simulink model "MyBattery_RTW"  (Simulink 10.1)
settings: Solver=ode1  StartTime=0.0  StopTime=inf  FixedStep=0.0002  RelTol=1e-3
PreLoadFcn:
  | vehicle = 'Car'; if ~length(which('cmself')), cmenv; end
  | MyBattery_RTW_bus
InitFcn:
  | vehicle = 'Car'; if ~length(which('cmself')), cmenv; end
  | MyBattery_RTW_bus
libraries: CarMaker4SL x2, simulink x1, simulink_need_slupdate x1
Description:
  | CarMaker Plug-in Model Target
settings Model: Creator=ml  LastModifiedBy=ml
settings DataIOCC: SaveFormat=Dataset  ReturnWorkspaceOutputs=on
settings OptimizationCC: LifeSpan=auto
settings DebuggingCC: UnderspecifiedInitializationDetection=Simplified  MergeDetectMultiDrivingBlocksExec=error  SFUnexpectedBacktrackingDiag=error  SFNoUnconditionalDefaultTransitionDiag=error  SFExecutionAtInitializationDiag=warning  ArithmeticOperatorsInVariantConditions=error
settings HardwareCC: ProdBitPerPointer=64  ProdBitPerSizeT=64  ProdBitPerPtrDiffT=64  ProdLargestAtomicFloat=Float  ProdIntDivRoundTo=Zero  ProdEndianess=LittleEndian  ProdWordSize=64  ProdHWDeviceType=Intel->x86-64 (Windows64)
settings ModelReferenceCC: PropagateSignalLabelsOutOfModel=on
settings SFSimCC: SimUseLocalCustomCode=on  CustomCodeUndefinedFunction=FilterOut
settings RTWCC: Description=CarMaker Plug-in Model Target  SystemTargetFile=CarMaker.tlc  TemplateMakefile=CarMaker_unix-win64.tmf  RTWUseLocalCustomCode=on
settings CodeAppCC: MaxIdLength=127  StateflowObjectComments=off
settings STFCustomTargetCC: TargetLangStandard=C99 (ISO)  CombineOutputUpdateFcns=on  MultiInstanceERTCode=on  CodeInterfacePackaging=Reusable function  GRTInterface=off  GenerateAllocFcn=on  SystemTargetFile=CarMaker.tlc
settings GRTTargetCC: TargetLangStandard=C99 (ISO)  ParMdlRefBuildCompliant=off  CompOptLevelCompliant=off  ConcurrentExecutionCompliant=off  CombineOutputUpdateFcns=on  MatFileLogging=off  MultiInstanceERTCode=on  CodeInterfacePackaging=Reusable function  CPPClassGenCompliant=off  GRTInterface=off  GenerateAllocFcn=on  UseToolchainInfoCompliant=off
settings CustomProperty: DataType=string
settings EnumStrPairs: String=Car
settings ConfigComp: CovMetricSettings=dwe  CovHtmlReporting=off  CovSaveCumulativeToWorkspaceVar=off  CovSaveSingleToWorkspaceVar=off  CovExternalEMLEnable=on

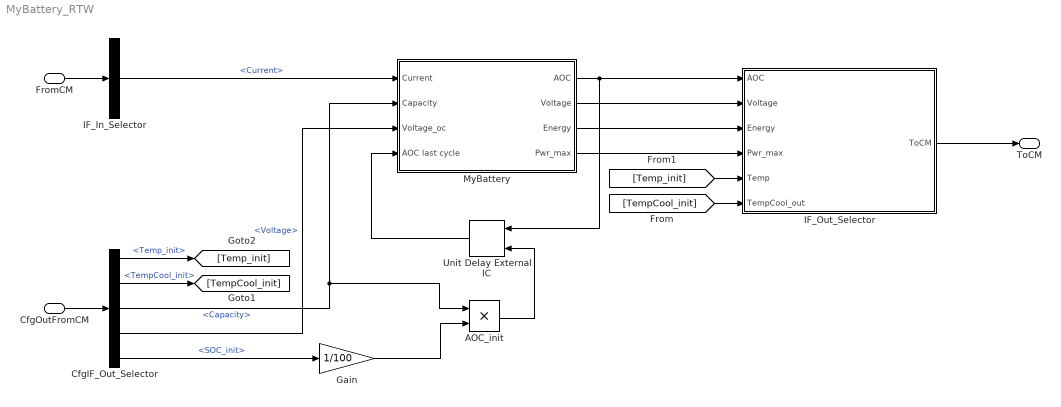
== system MyBattery_RTW ==
  FromCM : Inport  OutDataTypeStr=Bus: cmPTBatteryIn
  CfgOutFromCM : Inport  Port=2  OutDataTypeStr=Bus: cmPTBatteryCfgOut
  AOC_init : Product  RndMeth=Zero
  CfgIF_Out_Selector : BusSelector  OutputSignals=Temp_init,TempCool_init,Capacity,Voltage,SOC_init
  Gain : Gain  Gain=1/100
  IF_In_Selector : BusSelector  OutputSignals=Current
  IF_Out_Selector : Subsystem  mask(Signal Selection){}
      mask help: Signal Selection Block
      settings: OpenFcn=cmSignalSelect('SignalSelection_CB',gcb)
  MyBattery : Subsystem
  Unit Delay External IC : simulink_need_slupdate/Unit Delay External IC  tsamp=-1
      settings: SourceProductBaseCode=SL
  ToCM : Outport  OutDataTypeStr=Bus: cmPTBatteryOut
  wires:
  IF_Out_Selector/1(ToCM) -> ToCM/1
  MyBattery/3(Energy) -> IF_Out_Selector/3(Energy)
  Gain/1 -> AOC_init/2
  FromCM/1 -> IF_In_Selector/1
  CfgIF_Out_Selector/3 -> MyBattery/2(Capacity), AOC_init/1  "<Capacity>"
  CfgOutFromCM/1 -> CfgIF_Out_Selector/1
  [Temp_init] -> IF_Out_Selector/5(Temp)
  [TempCool_init] -> IF_Out_Selector/6(TempCool_out)
  MyBattery/4(Pwr_max) -> IF_Out_Selector/4(Pwr_max)
  CfgIF_Out_Selector/1 -> [Temp_init]  "<Temp_init>"
  Unit Delay External IC/1 -> MyBattery/4(AOC last cycle)
  CfgIF_Out_Selector/2 -> [TempCool_init]  "<TempCool_init>"
  CfgIF_Out_Selector/4 -> MyBattery/3(Voltage_oc)  "<Voltage>"
  IF_In_Selector/1 -> MyBattery/1(Current)  "<Current>"
  MyBattery/2(Voltage) -> IF_Out_Selector/2(Voltage)
  MyBattery/1(AOC) -> IF_Out_Selector/1(AOC), Unit Delay External IC/1
  AOC_init/1 -> Unit Delay External IC/2
  CfgIF_Out_Selector/5 -> Gain/1  "<SOC_init>"

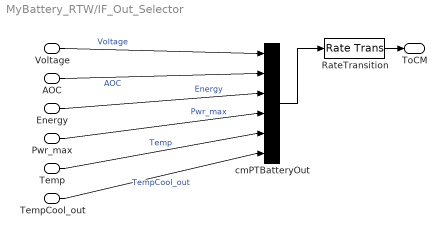
== system MyBattery_RTW/IF_Out_Selector ==
  AOC : Inport
  Voltage : Inport  Port=2
  Energy : Inport  Port=3
  Pwr_max : Inport  Port=4
  Temp : Inport  Port=5
  TempCool_out : Inport  Port=6
  RateTransition : RateTransition  OutPortSampleTime=str2num(get_param(bdroot,'FixedStep'))
  cmPTBatteryOut : BusCreator  Inputs=6
  ToCM : Outport
  wires:
  RateTransition/1 -> ToCM/1
  cmPTBatteryOut/1 -> RateTransition/1
  AOC/1 -> cmPTBatteryOut/2  "AOC"
  Voltage/1 -> cmPTBatteryOut/1  "Voltage"
  Energy/1 -> cmPTBatteryOut/3  "Energy"
  Pwr_max/1 -> cmPTBatteryOut/4  "Pwr_max"
  Temp/1 -> cmPTBatteryOut/5  "Temp"
  TempCool_out/1 -> cmPTBatteryOut/6  "TempCool_out"

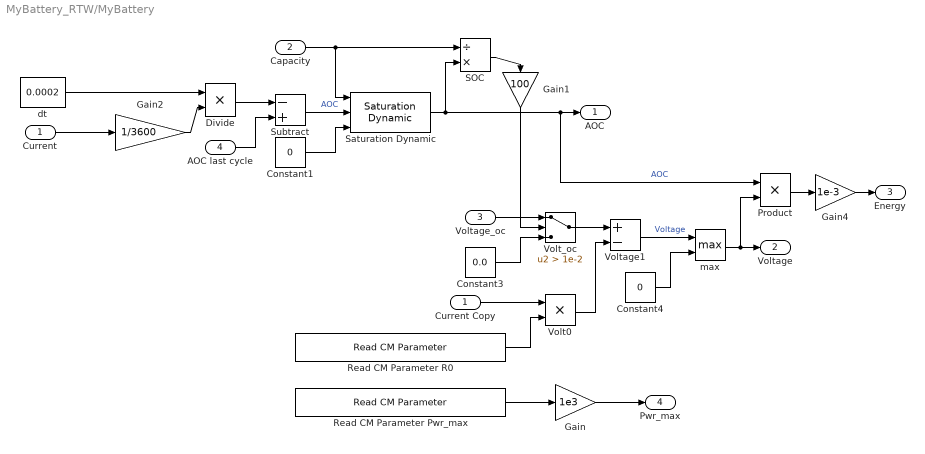
== system MyBattery_RTW/MyBattery ==
  Current : Inport
  Capacity : Inport  Port=2
  Voltage_oc : Inport  Port=3
  AOC last cycle : Inport  Port=4
  Constant1 : Constant  Value=0
  Constant3 : Constant  Value=0.0
  Constant4 : Constant  Value=0
  Current Copy : InportShadow
  Divide : Product  Inputs=**
  Gain : Gain  Gain=1e3
  Gain1 : Gain  Gain=100
  Gain2 : Gain  Gain=1/3600
  Gain4 : Gain  Gain=1e-3
  Product : Product  RndMeth=Zero
  Read CM Parameter Pwr_max : CarMaker4SL/Read CM Parameter  xfile=Vehicle  xkey=PowerTrain.PowerSupply.BattLV.Pwr_max  xnout=1  xdefaults=100  xmuxed=on  xstime=Continuous
      settings: SourceProductName=CarMaker4SL
  Read CM Parameter R0 : CarMaker4SL/Read CM Parameter  xfile=Vehicle  xkey=PowerTrain.PowerSupply.BattLV.R0  xnout=1  xdefaults=0.0012  xmuxed=on  xstime=Continuous
      settings: SourceProductName=CarMaker4SL
  SOC : Product  Inputs=/*
  Saturation Dynamic : simulink/Discontinuities/Saturation Dynamic  OutMin=[]  OutMax=[]  OutDataTypeStr=Inherit: Same as second input  OutDataType=sfix(16)  OutScaling=2^-10  DoSatur=off
  Subtract : Sum  Inputs=-+
  Volt0 : Product  RndMeth=Zero
  Volt_oc : Switch  Criteria=u2 > Threshold  Threshold=1e-2
  Voltage1 : Sum  Inputs=+-
  dt : Constant  Value=0.0002
  max : MinMax  Function=max  Inputs=2
  AOC : Outport  VectorParamsAs1DForOutWhenUnconnected=off
  Voltage : Outport  Port=2  VectorParamsAs1DForOutWhenUnconnected=off
  Energy : Outport  Port=3  VectorParamsAs1DForOutWhenUnconnected=off
  Pwr_max : Outport  Port=4  VectorParamsAs1DForOutWhenUnconnected=off
  wires:
  Saturation Dynamic/1 -> AOC/1, Product/1, SOC/2  "AOC"
  Divide/1 -> Subtract/1
  dt/1 -> Divide/1
  Subtract/1 -> Saturation Dynamic/2  "AOC"
  Constant1/1 -> Saturation Dynamic/3
  Capacity/1 -> Saturation Dynamic/1, SOC/1
  Read CM Parameter Pwr_max/1 -> Gain/1
  SOC/1 -> Gain1/1
  Voltage_oc/1 -> Volt_oc/1
  Constant3/1 -> Volt_oc/3
  Read CM Parameter R0/1 -> Volt0/2
  Volt_oc/1 -> Voltage1/1
  Volt0/1 -> Voltage1/2
  Voltage1/1 -> max/1  "Voltage"
  Constant4/1 -> max/2
  max/1 -> Voltage/1, Product/2
  Product/1 -> Gain4/1
  Gain/1 -> Pwr_max/1
  AOC last cycle/1 -> Subtract/2
  Gain2/1 -> Divide/2
  Gain1/1 -> Volt_oc/2
  Current/1 -> Gain2/1
  Current Copy/1 -> Volt0/1
  Gain4/1 -> Energy/1
